simulink model "bici_v2"  (R2013a)
settings: Solver=ode3  SolverMode=SingleTasking  StartTime=0.0  StopTime=10.0  RelTol=1e-3
PreLoadFcn:
  | waijung.modelPreload; % Required for working with Waijung Blockset. Do not remove.
undefined symbols (not defined in the file or in its folder): HSEOSC, Link, LQFP176, ST, STM32F417IG
libraries: simulink x6, stm32f4_tim_lib x6, stm32f4_io_lib x2, stm32f4_adc_lib x1, stm32f4_device_config_lib x1
(part 1 of 2)
CloseFcn:
  | waijung.modelClose; % Required for working with Waijung Blockset. Do not remove.
settings Model: Creator=Juan Esteban  LastModifiedBy=Juan Esteban
settings OptimizationCC: OptimizeModelRefInitCode=on  LifeSpan=1
settings HardwareCC: ProdEndianess=LittleEndian  ProdHWDeviceType=ARM Compatible->Cortex - M4  TargetEndianess=LittleEndian  TargetHWDeviceType=ARM Compatible->Cortex - M4
settings RTWCC: SystemTargetFile=stm32f4.tlc  GenerateMakefile=off  TemplateMakefile=ert_default_tmf  Description=STM32F4 Target  ProcessScript=stm32f4_make_rtw_hook
settings CodeAppCC: IgnoreCustomStorageClasses=off
settings STFCustomTargetCC: ModelReferenceCompliant=off  CombineOutputUpdateFcns=on  ERTCustomFileBanners=on  SupportNonInlinedSFcns=off  MATLABClassNameForMDSCustomization=Simulink.SoftwareTarget.ERTCustomization  SystemTargetFile=stm32f4.tlc
settings ERTTargetCC: GenerateSampleERTMain=off  ModelReferenceCompliant=off  ParMdlRefBuildCompliant=off  CompOptLevelCompliant=off  ConcurrentExecutionCompliant=off  ERTFirstTimeCompliant=off  SupportContinuousTime=on  ModelStepFunctionPrototypeControlCompliant=off  CPPClassGenCompliant=off  ERTSrcFileBannerTemplate=stm32f4_code_template.cgt  ERTHdrFileBannerTemplate=stm32f4_code_template.cgt  ERTDataSrcFileTemplate=stm32f4_code_template.cgt  ERTDataHdrFileTemplate=stm32f4_code_template.cgt  ERTCustomFileTemplate=stm32f4_file_process.tlc

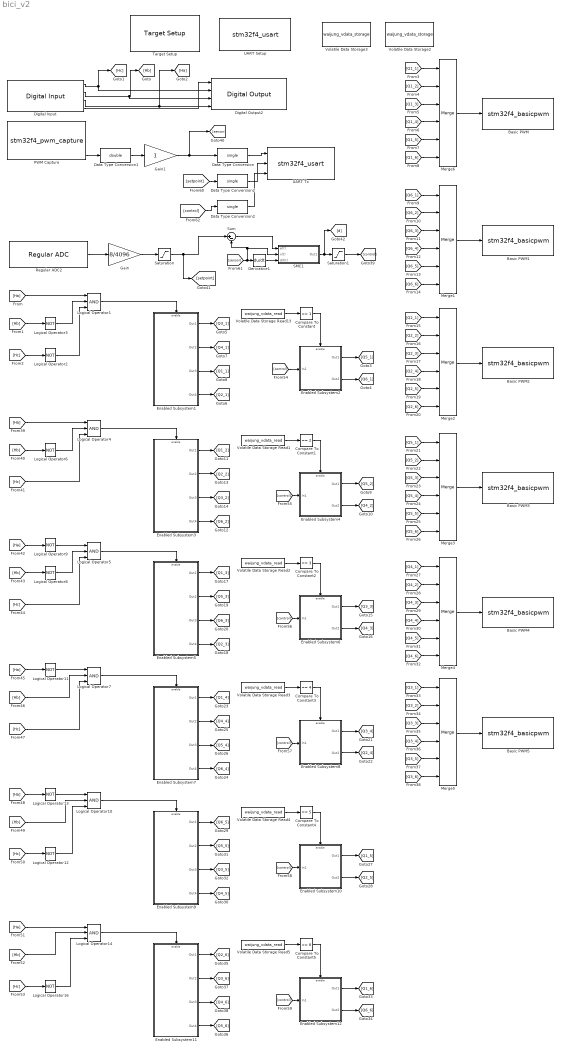
== system bici_v2 ==
  Basic PWM : S-Function  FunctionName=stm32f4_basicpwm  Parameters=timer,pwmperiod,ch1pin,ch2pin,ch3pin,ch4pin,sampletime,sampletimestr,blockid,apb,portstr,pinstr,pinmat,timarr,timprescale,chmat,polaritystr  EnableBusSupport=off  mask(stm32f4_basicpwm){timer=3, pwmperiod=2e-4, polarity=Active High, polaritystr=TIM_OCPolarity_High, ch1pin=A6, ch2pin=Not available - Do not use, ch3pin=Not available - Do not use, ch4pin=Not available - Do not use, sampletime=0.01, sampletimestr=0.01, blockid=BasicPWM, portpinstr=A6,,,, enablecustomportlabel=off, cinputportlabel=In1, In2, In3, In4, coutputportlabel=0, apb=1, portstr=["A"], pinstr=["GPIO_Pin_6"], pinmat=[1 6], timarr=16799, timprescale=0, chmat=[1]}
      mask prompts: pwmperiod "PWM Period (seconds)"; ch1pin "Channel 1"; ch2pin "Channel 2"; ch3pin "Channel 3"; ch4pin "Channel 4"; sampletime "Sample time (sec)"; sampletimestr "Compiled sample time (sec) in string"; portpinstr "Port pin string"; enablecustomportlabel "Enable custom port labels"; cinputportlabel "Custom input port labels (Ex. In1, In2, In3)"; coutputportlabel "Custom output port labels (Ex. Out1, Out2, Out3)"; portstr "Port string"; pinstr "Pin string"; pinmat "Pin matrix"; timarr "Timer ARR"; timprescale "Timer PRESCALE"; chmat "Channel order"
      mask help:
      | This block implements basic Edge-aligned Pulse Width Modulation (PWM) generation.
      | All timers are 16-bit. The PWM period is fixed (per timer).
      mask init:
      | stm32f4_basicpwm_callback('init');
      mask Help: web(fullfile(waijungdocroot,'stm32f4_basicpwm.htm'),'-browser')
      mask TypeOptions timer: 1 | 2 | 3 | 4 | 5 | 8 | 9 | 10 | 11 | 12 | 13 | 14
      mask Callback timer: stm32f4_basicpwm_callback('timer');
      mask Callback pwmperiod: stm32f4_basicpwm_callback('pwmperiod');
      mask TypeOptions polarity: Active High | Active Low
      mask Callback polarity: stm32f4_basicpwm_callback('polarity');
      mask TypeOptions ch1pin: Not available - Do not use | A6 | B4 | C6
      mask Callback ch1pin: stm32f4_basicpwm_callback('ch1pin');
      mask TypeOptions ch2pin: Not available - Do not use | A7 | B5 | C7
      mask Callback ch2pin: stm32f4_basicpwm_callback('ch2pin');
      mask TypeOptions ch3pin: Not available - Do not use | B0 | C8
      mask Callback ch3pin: stm32f4_basicpwm_callback('ch3pin');
      mask TypeOptions ch4pin: Not available - Do not use | B1 | C9
      mask Callback ch4pin: stm32f4_basicpwm_callback('ch4pin');
      mask Callback sampletime: stm32f4_basicpwm_callback('sampletime');
      mask Callback sampletimestr: stm32f4_basicpwm_callback('sampletimestr');
      mask Callback blockid: stm32f4_basicpwm_callback('blockid');
      mask Callback enablecustomportlabel: stm32f4_basicpwm_callback('enablecustomportlabel');
      mask Display: text(0.95, 0.5, 'Timer: 3\nPolarity: Active High\nPeriod (sec) 2e-4\nTs (sec): 0.01','ver','middle','hor','right');port_label('input', 1,'CH1 (A6)')
  Basic PWM1 : S-Function  FunctionName=stm32f4_basicpwm  Parameters=timer,pwmperiod,ch1pin,ch2pin,ch3pin,ch4pin,sampletime,sampletimestr,blockid,apb,portstr,pinstr,pinmat,timarr,timprescale,chmat,polaritystr  EnableBusSupport=off  mask(stm32f4_basicpwm){timer=4, pwmperiod=2e-4, polarity=Active High, polaritystr=TIM_OCPolarity_High, ch1pin=B6, ch2pin=Not available - Do not use, ch3pin=Not available - Do not use, ch4pin=Not available - Do not use, sampletime=0.01, sampletimestr=0.01, blockid=BasicPWM1, portpinstr=B6,,,, enablecustomportlabel=off, cinputportlabel=In1, In2, In3, In4, coutputportlabel=0, apb=1, portstr=["B"], pinstr=["GPIO_Pin_6"], pinmat=[1 6], timarr=16799, timprescale=0, chmat=[1]}
      mask prompts: pwmperiod "PWM Period (seconds)"; ch1pin "Channel 1"; ch2pin "Channel 2"; ch3pin "Channel 3"; ch4pin "Channel 4"; sampletime "Sample time (sec)"; sampletimestr "Compiled sample time (sec) in string"; portpinstr "Port pin string"; enablecustomportlabel "Enable custom port labels"; cinputportlabel "Custom input port labels (Ex. In1, In2, In3)"; coutputportlabel "Custom output port labels (Ex. Out1, Out2, Out3)"; portstr "Port string"; pinstr "Pin string"; pinmat "Pin matrix"; timarr "Timer ARR"; timprescale "Timer PRESCALE"; chmat "Channel order"
      mask help:
      | This block implements basic Edge-aligned Pulse Width Modulation (PWM) generation.
      | All timers are 16-bit. The PWM period is fixed (per timer).
      mask init:
      | stm32f4_basicpwm_callback('init');
      mask Help: web(fullfile(waijungdocroot,'stm32f4_basicpwm.htm'),'-browser')
      mask TypeOptions timer: 1 | 2 | 3 | 4 | 5 | 8 | 9 | 10 | 11 | 12 | 13 | 14
      mask Callback timer: stm32f4_basicpwm_callback('timer');
      mask Callback pwmperiod: stm32f4_basicpwm_callback('pwmperiod');
      mask TypeOptions polarity: Active High | Active Low
      mask Callback polarity: stm32f4_basicpwm_callback('polarity');
      mask TypeOptions ch1pin: Not available - Do not use | B6 | D12
      mask Callback ch1pin: stm32f4_basicpwm_callback('ch1pin');
      mask TypeOptions ch2pin: Not available - Do not use | B7 | D13
      mask Callback ch2pin: stm32f4_basicpwm_callback('ch2pin');
      mask TypeOptions ch3pin: Not available - Do not use | B8 | D14
      mask Callback ch3pin: stm32f4_basicpwm_callback('ch3pin');
      mask TypeOptions ch4pin: Not available - Do not use | B9 | D15
      mask Callback ch4pin: stm32f4_basicpwm_callback('ch4pin');
      mask Callback sampletime: stm32f4_basicpwm_callback('sampletime');
      mask Callback sampletimestr: stm32f4_basicpwm_callback('sampletimestr');
      mask Callback blockid: stm32f4_basicpwm_callback('blockid');
      mask Callback enablecustomportlabel: stm32f4_basicpwm_callback('enablecustomportlabel');
      mask Display: text(0.95, 0.5, 'Timer: 4\nPolarity: Active High\nPeriod (sec) 2e-4\nTs (sec): 0.01','ver','middle','hor','right');port_label('input', 1,'CH1 (B6)')
  Basic PWM2 : S-Function  FunctionName=stm32f4_basicpwm  Parameters=timer,pwmperiod,ch1pin,ch2pin,ch3pin,ch4pin,sampletime,sampletimestr,blockid,apb,portstr,pinstr,pinmat,timarr,timprescale,chmat,polaritystr  EnableBusSupport=off  mask(stm32f4_basicpwm){timer=1, pwmperiod=2e-4, polarity=Active High, polaritystr=TIM_OCPolarity_High, ch1pin=A8, ch2pin=Not available - Do not use, ch3pin=Not available - Do not use, ch4pin=Not available - Do not use, sampletime=0.01, sampletimestr=0.01, blockid=BasicPWM2, portpinstr=A8,,,, enablecustomportlabel=off, cinputportlabel=In1, In2, In3, In4, coutputportlabel=0, apb=2, portstr=["A"], pinstr=["GPIO_Pin_8"], pinmat=[1 8], timarr=33599, timprescale=0, chmat=[1]}
      mask prompts: pwmperiod "PWM Period (seconds)"; ch1pin "Channel 1"; ch2pin "Channel 2"; ch3pin "Channel 3"; ch4pin "Channel 4"; sampletime "Sample time (sec)"; sampletimestr "Compiled sample time (sec) in string"; portpinstr "Port pin string"; enablecustomportlabel "Enable custom port labels"; cinputportlabel "Custom input port labels (Ex. In1, In2, In3)"; coutputportlabel "Custom output port labels (Ex. Out1, Out2, Out3)"; portstr "Port string"; pinstr "Pin string"; pinmat "Pin matrix"; timarr "Timer ARR"; timprescale "Timer PRESCALE"; chmat "Channel order"
      mask help:
      | This block implements basic Edge-aligned Pulse Width Modulation (PWM) generation.
      | All timers are 16-bit. The PWM period is fixed (per timer).
      mask init:
      | stm32f4_basicpwm_callback('init');
      mask Help: web(fullfile(waijungdocroot,'stm32f4_basicpwm.htm'),'-browser')
      mask TypeOptions timer: 1 | 2 | 3 | 4 | 5 | 8 | 9 | 10 | 11 | 12 | 13 | 14
      mask Callback timer: stm32f4_basicpwm_callback('timer');
      mask Callback pwmperiod: stm32f4_basicpwm_callback('pwmperiod');
      mask TypeOptions polarity: Active High | Active Low
      mask Callback polarity: stm32f4_basicpwm_callback('polarity');
      mask TypeOptions ch1pin: Not available - Do not use | A8 | E9
      mask Callback ch1pin: stm32f4_basicpwm_callback('ch1pin');
      mask TypeOptions ch2pin: Not available - Do not use | A9 | E11
      mask Callback ch2pin: stm32f4_basicpwm_callback('ch2pin');
      mask TypeOptions ch3pin: Not available - Do not use | A10 | E13
      mask Callback ch3pin: stm32f4_basicpwm_callback('ch3pin');
      mask TypeOptions ch4pin: Not available - Do not use | A11 | E14
      mask Callback ch4pin: stm32f4_basicpwm_callback('ch4pin');
      mask Callback sampletime: stm32f4_basicpwm_callback('sampletime');
      mask Callback sampletimestr: stm32f4_basicpwm_callback('sampletimestr');
      mask Callback blockid: stm32f4_basicpwm_callback('blockid');
      mask Callback enablecustomportlabel: stm32f4_basicpwm_callback('enablecustomportlabel');
      mask Display: text(0.95, 0.5, 'Timer: 1\nPolarity: Active High\nPeriod (sec) 2e-4\nTs (sec): 0.01','ver','middle','hor','right');port_label('input', 1,'CH1 (A8)')
  Basic PWM3 : S-Function  FunctionName=stm32f4_basicpwm  Parameters=timer,pwmperiod,ch1pin,ch2pin,ch3pin,ch4pin,sampletime,sampletimestr,blockid,apb,portstr,pinstr,pinmat,timarr,timprescale,chmat,polaritystr  EnableBusSupport=off  mask(stm32f4_basicpwm){timer=2, pwmperiod=2e-4, polarity=Active High, polaritystr=TIM_OCPolarity_High, ch1pin=A0, ch2pin=Not available - Do not use, ch3pin=Not available - Do not use, ch4pin=Not available - Do not use, sampletime=0.01, sampletimestr=0.01, blockid=BasicPWM3, portpinstr=A0,,,, enablecustomportlabel=off, cinputportlabel=In1, In2, In3, In4, coutputportlabel=0, apb=1, portstr=["A"], pinstr=["GPIO_Pin_0"], pinmat=[1 0], timarr=16799, timprescale=0, chmat=[1]}
      mask prompts: pwmperiod "PWM Period (seconds)"; ch1pin "Channel 1"; ch2pin "Channel 2"; ch3pin "Channel 3"; ch4pin "Channel 4"; sampletime "Sample time (sec)"; sampletimestr "Compiled sample time (sec) in string"; portpinstr "Port pin string"; enablecustomportlabel "Enable custom port labels"; cinputportlabel "Custom input port labels (Ex. In1, In2, In3)"; coutputportlabel "Custom output port labels (Ex. Out1, Out2, Out3)"; portstr "Port string"; pinstr "Pin string"; pinmat "Pin matrix"; timarr "Timer ARR"; timprescale "Timer PRESCALE"; chmat "Channel order"
      mask help:
      | This block implements basic Edge-aligned Pulse Width Modulation (PWM) generation.
      | All timers are 16-bit. The PWM period is fixed (per timer).
      mask init:
      | stm32f4_basicpwm_callback('init');
      mask Help: web(fullfile(waijungdocroot,'stm32f4_basicpwm.htm'),'-browser')
      mask TypeOptions timer: 1 | 2 | 3 | 4 | 5 | 8 | 9 | 10 | 11 | 12 | 13 | 14
      mask Callback timer: stm32f4_basicpwm_callback('timer');
      mask Callback pwmperiod: stm32f4_basicpwm_callback('pwmperiod');
      mask TypeOptions polarity: Active High | Active Low
      mask Callback polarity: stm32f4_basicpwm_callback('polarity');
      mask TypeOptions ch1pin: Not available - Do not use | A0 | A5 | A15
      mask Callback ch1pin: stm32f4_basicpwm_callback('ch1pin');
      mask TypeOptions ch2pin: Not available - Do not use | A1 | B3
      mask Callback ch2pin: stm32f4_basicpwm_callback('ch2pin');
      mask TypeOptions ch3pin: Not available - Do not use | A2 | B10
      mask Callback ch3pin: stm32f4_basicpwm_callback('ch3pin');
      mask TypeOptions ch4pin: Not available - Do not use | A3 | B11
      mask Callback ch4pin: stm32f4_basicpwm_callback('ch4pin');
      mask Callback sampletime: stm32f4_basicpwm_callback('sampletime');
      mask Callback sampletimestr: stm32f4_basicpwm_callback('sampletimestr');
      mask Callback blockid: stm32f4_basicpwm_callback('blockid');
      mask Callback enablecustomportlabel: stm32f4_basicpwm_callback('enablecustomportlabel');
      mask Display: text(0.95, 0.5, 'Timer: 2\nPolarity: Active High\nPeriod (sec) 2e-4\nTs (sec): 0.01','ver','middle','hor','right');port_label('input', 1,'CH1 (A0)')
  Basic PWM4 : S-Function  FunctionName=stm32f4_basicpwm  Parameters=timer,pwmperiod,ch1pin,ch2pin,ch3pin,ch4pin,sampletime,sampletimestr,blockid,apb,portstr,pinstr,pinmat,timarr,timprescale,chmat,polaritystr  EnableBusSupport=off  mask(stm32f4_basicpwm){timer=5, pwmperiod=2e-4, polarity=Active High, polaritystr=TIM_OCPolarity_High, ch1pin=Not available - Do not use, ch2pin=A1, ch3pin=Not available - Do not use, ch4pin=Not available - Do not use, sampletime=0.01, sampletimestr=0.01, blockid=BasicPWM4, portpinstr=,A1,,, enablecustomportlabel=off, cinputportlabel=In1, In2, In3, In4, coutputportlabel=0, apb=1, portstr=["A"], pinstr=["GPIO_Pin_1"], pinmat=[1 1], timarr=16799, timprescale=0, chmat=[2]}
      mask prompts: pwmperiod "PWM Period (seconds)"; ch1pin "Channel 1"; ch2pin "Channel 2"; ch3pin "Channel 3"; ch4pin "Channel 4"; sampletime "Sample time (sec)"; sampletimestr "Compiled sample time (sec) in string"; portpinstr "Port pin string"; enablecustomportlabel "Enable custom port labels"; cinputportlabel "Custom input port labels (Ex. In1, In2, In3)"; coutputportlabel "Custom output port labels (Ex. Out1, Out2, Out3)"; portstr "Port string"; pinstr "Pin string"; pinmat "Pin matrix"; timarr "Timer ARR"; timprescale "Timer PRESCALE"; chmat "Channel order"
      mask help:
      | This block implements basic Edge-aligned Pulse Width Modulation (PWM) generation.
      | All timers are 16-bit. The PWM period is fixed (per timer).
      mask init:
      | stm32f4_basicpwm_callback('init');
      mask Help: web(fullfile(waijungdocroot,'stm32f4_basicpwm.htm'),'-browser')
      mask TypeOptions timer: 1 | 2 | 3 | 4 | 5 | 8 | 9 | 10 | 11 | 12 | 13 | 14
      mask Callback timer: stm32f4_basicpwm_callback('timer');
      mask Callback pwmperiod: stm32f4_basicpwm_callback('pwmperiod');
      mask TypeOptions polarity: Active High | Active Low
      mask Callback polarity: stm32f4_basicpwm_callback('polarity');
      mask TypeOptions ch1pin: Not available - Do not use | A0 | H10
      mask Callback ch1pin: stm32f4_basicpwm_callback('ch1pin');
      mask TypeOptions ch2pin: Not available - Do not use | A1 | H11
      mask Callback ch2pin: stm32f4_basicpwm_callback('ch2pin');
      mask TypeOptions ch3pin: Not available - Do not use | A2 | H12
      mask Callback ch3pin: stm32f4_basicpwm_callback('ch3pin');
      mask TypeOptions ch4pin: Not available - Do not use | A3 | I0
      mask Callback ch4pin: stm32f4_basicpwm_callback('ch4pin');
      mask Callback sampletime: stm32f4_basicpwm_callback('sampletime');
      mask Callback sampletimestr: stm32f4_basicpwm_callback('sampletimestr');
      mask Callback blockid: stm32f4_basicpwm_callback('blockid');
      mask Callback enablecustomportlabel: stm32f4_basicpwm_callback('enablecustomportlabel');
      mask Display: text(0.95, 0.5, 'Timer: 5\nPolarity: Active High\nPeriod (sec) 2e-4\nTs (sec): 0.01','ver','middle','hor','right');port_label('input', 1,'CH2 (A1)')
  Basic PWM5 : S-Function  FunctionName=stm32f4_basicpwm  Parameters=timer,pwmperiod,ch1pin,ch2pin,ch3pin,ch4pin,sampletime,sampletimestr,blockid,apb,portstr,pinstr,pinmat,timarr,timprescale,chmat,polaritystr  EnableBusSupport=off  mask(stm32f4_basicpwm){timer=9, pwmperiod=2e-4, polarity=Active High, polaritystr=TIM_OCPolarity_High, ch1pin=A2, ch2pin=Not available - Do not use, ch3pin=Not available - Do not use, ch4pin=Not available - Do not use, sampletime=0.01, sampletimestr=0.01, blockid=BasicPWM5, portpinstr=A2,,,, enablecustomportlabel=off, cinputportlabel=In1, In2, In3, In4, coutputportlabel=0, apb=2, portstr=["A"], pinstr=["GPIO_Pin_2"], pinmat=[1 2], timarr=33599, timprescale=0, chmat=[1]}
      mask prompts: pwmperiod "PWM Period (seconds)"; ch1pin "Channel 1"; ch2pin "Channel 2"; ch3pin "Channel 3"; ch4pin "Channel 4"; sampletime "Sample time (sec)"; sampletimestr "Compiled sample time (sec) in string"; portpinstr "Port pin string"; enablecustomportlabel "Enable custom port labels"; cinputportlabel "Custom input port labels (Ex. In1, In2, In3)"; coutputportlabel "Custom output port labels (Ex. Out1, Out2, Out3)"; portstr "Port string"; pinstr "Pin string"; pinmat "Pin matrix"; timarr "Timer ARR"; timprescale "Timer PRESCALE"; chmat "Channel order"
      mask help:
      | This block implements basic Edge-aligned Pulse Width Modulation (PWM) generation.
      | All timers are 16-bit. The PWM period is fixed (per timer).
      mask init:
      | stm32f4_basicpwm_callback('init');
      mask Help: web(fullfile(waijungdocroot,'stm32f4_basicpwm.htm'),'-browser')
      mask TypeOptions timer: 1 | 2 | 3 | 4 | 5 | 8 | 9 | 10 | 11 | 12 | 13 | 14
      mask Callback timer: stm32f4_basicpwm_callback('timer');
      mask Callback pwmperiod: stm32f4_basicpwm_callback('pwmperiod');
      mask TypeOptions polarity: Active High | Active Low
      mask Callback polarity: stm32f4_basicpwm_callback('polarity');
      mask TypeOptions ch1pin: Not available - Do not use | A2 | E5
      mask Callback ch1pin: stm32f4_basicpwm_callback('ch1pin');
      mask TypeOptions ch2pin: Not available - Do not use | A3 | E6
      mask Callback ch2pin: stm32f4_basicpwm_callback('ch2pin');
      mask TypeOptions ch3pin: Not available - Do not use
      mask Callback ch3pin: stm32f4_basicpwm_callback('ch3pin');
      mask TypeOptions ch4pin: Not available - Do not use
      mask Callback ch4pin: stm32f4_basicpwm_callback('ch4pin');
      mask Callback sampletime: stm32f4_basicpwm_callback('sampletime');
      mask Callback sampletimestr: stm32f4_basicpwm_callback('sampletimestr');
      mask Callback blockid: stm32f4_basicpwm_callback('blockid');
      mask Callback enablecustomportlabel: stm32f4_basicpwm_callback('enablecustomportlabel');
      mask Display: text(0.95, 0.5, 'Timer: 9\nPolarity: Active High\nPeriod (sec) 2e-4\nTs (sec): 0.01','ver','middle','hor','right');port_label('input', 1,'CH1 (A2)')
  Compare To Constant : simulink/Logic and Bit Operations/Compare To Constant  relop===  const=1  OutDataTypeStr=boolean
  Compare To Constant1 : simulink/Logic and Bit Operations/Compare To Constant  relop===  const=2  OutDataTypeStr=boolean
  Compare To Constant2 : simulink/Logic and Bit Operations/Compare To Constant  relop===  const=3  OutDataTypeStr=boolean
  Compare To Constant3 : simulink/Logic and Bit Operations/Compare To Constant  relop===  const=4  OutDataTypeStr=boolean
  Compare To Constant4 : simulink/Logic and Bit Operations/Compare To Constant  relop===  const=5  OutDataTypeStr=boolean
  Compare To Constant5 : simulink/Logic and Bit Operations/Compare To Constant  relop===  const=6  OutDataTypeStr=boolean
  Data Type Conversion : DataTypeConversion  OutDataTypeStr=single
  Data Type Conversion1 : DataTypeConversion  OutDataTypeStr=double
  Data Type Conversion2 : DataTypeConversion  OutDataTypeStr=single
  "Data Type Conversion2 " : DataTypeConversion  OutDataTypeStr=single
  Derivative1 : Derivative  CoefficientInTFapproximation=0
  Digital Input : stm32f4_io_lib/Digital Input  port=D  speed=100  porttype=Pull Up  porttypestr=UP  use_pin0=on  use_pin1=on  use_pin2=on  use_pin3=on  use_pin4=off  use_pin5=off  use_pin6=off  use_pin7=off  use_pin8=off  use_pin9=off  use_pin10=off  use_pin11=off  use_pin12=off  use_pin13=off  use_pin14=off  use_pin15=off  pinstr=GPIO_Pin_0 | GPIO_Pin_1 | GPIO_Pin_2 | GPIO_Pin_3  usedpinarray="[1  1  1  1  0  0  0  0  0  0  0  0  0  0  0  0]"  bitbandingstr=|  sampletime=-1  sampletimestr=0.01  blockid=DigitalInput  enablecustomportlabel=off  glabalinit=off  cinputportlabel=In1, In2  coutputportlabel=Out1, Out2
      | #define DigitalInput_D0 Peripheral_BB(GPIOD->IDR, 0)  /* Output pin */
      | #define DigitalInput_D1 Peripheral_BB(GPIOD->IDR, 1)  /* Output pin */
      | #define DigitalInput_D2 Peripheral_BB(GPIOD->IDR, 2)  /* Output pin */
      | #define DigitalInput_D3 Peripheral_BB(GPIOD->IDR, 3)  /* Output pin */
  Digital Output2 : stm32f4_io_lib/Digital Output  use_bitband=on  port=D  speed=100  porttype=Push Pull  porttypestr=PP  use_pin0=off  use_pin1=off  use_pin2=off  use_pin3=off  use_pin4=off  use_pin5=off  use_pin6=off  use_pin7=off  use_pin8=off  use_pin9=off  use_pin10=off  use_pin11=off  use_pin12=on  use_pin13=on  use_pin14=on  use_pin15=on  pinstr=GPIO_Pin_12 | GPIO_Pin_13 | GPIO_Pin_14 | GPIO_Pin_15  usedpinarray="[0  0  0  0  0  0  0  0  0  0  0  0  1  1  1  1]"  bitbandingstr=|  sampletime=-1  sampletimestr=0.01  blockid=DigitalOutput2  enablecustomportlabel=off  globalinit=off  cinputportlabel=In1, In2  coutputportlabel=0
      | #define DigitalOutput2_D12 Peripheral_BB(GPIOD->ODR, 12)  /* Output pin */
      | #define DigitalOutput2_D13 Peripheral_BB(GPIOD->ODR, 13)  /* Output pin */
      | #define DigitalOutput2_D14 Peripheral_BB(GPIOD->ODR, 14)  /* Output pin */
      | #define DigitalOutput2_D15 Peripheral_BB(GPIOD->ODR, 15)  /* Output pin */
  Enabled Subsystem1 : Subsystem  TreatAsAtomicUnit=on
  Enabled Subsystem10 : Subsystem  TreatAsAtomicUnit=on
  Enabled Subsystem11 : Subsystem  TreatAsAtomicUnit=on
  Enabled Subsystem12 : Subsystem  TreatAsAtomicUnit=on
  Enabled Subsystem2 : Subsystem  TreatAsAtomicUnit=on
  Enabled Subsystem3 : Subsystem  TreatAsAtomicUnit=on
  Enabled Subsystem4 : Subsystem  TreatAsAtomicUnit=on
  Enabled Subsystem5 : Subsystem  TreatAsAtomicUnit=on
  Enabled Subsystem6 : Subsystem  TreatAsAtomicUnit=on
  Enabled Subsystem7 : Subsystem  TreatAsAtomicUnit=on
  Enabled Subsystem8 : Subsystem  TreatAsAtomicUnit=on
  Enabled Subsystem9 : Subsystem  TreatAsAtomicUnit=on
  Gain : Gain  Gain=8/4096
  Gain1 : Gain
  Logical Operator{1,4..5,7,10,14} (6 alike) : Logic  Inputs=3  AllPortsSameDT=off  OutDataTypeStr=boolean
  Logical Operator{2..3,6,8..9,11..13,16} (9 alike) : Logic  Operator=NOT  Inputs=3  AllPortsSameDT=off  OutDataTypeStr=boolean
  Merge{1..6} (6 alike) : Merge  Inputs=6
  PWM Capture : S-Function  FunctionName=stm32f4_pwm_capture  Parameters=conf,inputporttype,inputportwidth,outputporttype,outputportwidth,optionstring,sampletime,blockid  EnableBusSupport=off  mask(stm32f4_pwm_capture){conf=Capture, timer=8, lasttimer=8, pin=C7, pintype=Pull Up, edge=Rising, datatype=single, portpinstr=0, sampletime=inf, blockid=PWMCapture, inputporttype=[], inputportwidth=[], inputportlabel={}, outputporttype=[3 1 1 1], outputportwidth=[], outputportlabel={'READY','+Width (sec)','+Duty (%)','Frequency (Hz)'}, compat=0, optionstring=["8","2","C","7","2","16","Rising","UP","float"]}
      mask prompts: conf "Configuration"; lasttimer "Last Timer"; pin "Capture Pin"; pintype "Capture Pin Type (Pull-Up/Pull-Down)"; edge "Capture Edge"; datatype "Output data type"; portpinstr "Port Pin String"; sampletime "Sample time (sec)"; blockid "Block ID"; inputporttype "Input Port Type"; inputportwidth "Input Port Width"; inputportlabel "Input Port Label"; outputporttype "Output Port Type"; outputportwidth "Output Port Width"; outputportlabel "Output port label"; compat "Compatibility (Reserved for future use)"; optionstring "String(s) to be passed to TLC"
      mask help:
      | Capture Edge:
      |  Rising - PWM period start from rising edge of pulse N to rising edge of pulse N+1
      |  Falling - PWM period start from falling edge of pulse N to falling edge of pulse N+1
      | Capture data type:
      |  Capture data type, selectable to double or single.
      |
      | Output:
      |  READY - indicate the status of capture, a non-zero value indicate data is ready.
      |  +Width - positive pulse width, in unit of second.
      |  +Duty - positive duty cycle, 0 to 100%
      |  Frequency - signal frequency in unit of Hz
      |
      | Note: caprure period should not longer than 1 second (Maximum limit is 3 seconds)
      mask init:
      | stm32f4_pwm_capture_callback('init');
      mask Help: web(fullfile(waijungdocroot,'stm32f4_pwm_capture.htm'), '-browser')
      mask TypeOptions conf: Capture
      mask Callback conf: stm32f4_pwm_capture_callback('conf');
      mask TypeOptions timer: 1 | 2 | 3 | 4 | 5 | 8
      mask Callback timer: stm32f4_pwm_capture_callback('timer');
      mask TypeOptions pin: Not used | C6 | I5 | C7 | I6 | C8 | I7 | C9 | I2
      mask TypeOptions pintype: None | Pull Up | Pull Down
      mask TypeOptions edge: Rising | Falling
      mask TypeOptions datatype: double | single
      mask Callback sampletime: stm32f4_pwm_capture_callback('sampletime');
      mask Callback blockid: stm32f4_pwm_capture_callback('blockid');
      mask Display: text(0.05, 0.5, 'Timer: 8 (16 bit)\nInput Pin: C7\nEdge: Rising\nTs (sec): 0.01','ver','middle','hor','left'); port_label('output', 1,'READY'); port_label('output', 2,'+Width (sec)'); port_label('output', 3,'+Duty (%)'); port_label('output', 4,'Frequency (Hz)');
  Regular ADC2 : stm32f4_adc_lib/Regular ADC  adcmodule=1  outputdatatype=Double  prescaler=2  prescalerstr=ADC_Prescaler_Div2  chsamplingtime=Auto  chsamplingtimestr=ADC_SampleTime_480Cycles  read_an0=off  read_an1=off  read_an2=off  read_an3=off  read_an4=off  read_an5=off  read_an6=off  read_an7=off  read_an8=off  read_an9=off  read_an10=on  read_an11=off  read_an12=off  read_an13=off  read_an14=off  read_an15=off  read_an16=off  read_an17=off  read_an18=off  pinstr=GPIO_Pin_10  usedpinarray="[0  0  0  0  0  0  0  0  0  0  1  0  0  0  0  0  0  0  0]"  usedportidarray=[2]  usedpinidarray=[0]  usedpinidcount=1  sampletime=-1  blockid=RegularADC2  enablecustomportlabel=off  cinputportlabel=0  coutputportlabel=Out1, Out2
  SMC1 : Subsystem  TreatAsAtomicUnit=on
  Saturation : Saturate  UpperLimit=8  LowerLimit=0
  Saturation1 : Saturate  UpperLimit=60  LowerLimit=0
  Sum : Sum  Inputs=|+-
  Target Setup : stm32f4_device_config_lib/Target Setup  Priority=100  compiler=GNU ARM  previous_compiler=GNU ARM  mcu=STM32F417IG (LQFP176)  mcustr=STM32F417IG  clockconfig=HSEOSC-8MHz  system_stm32f4xx_c_path=C:\waijung17_03a\targets\stm32f4_target\stm32f4\utils\system_stm32f4xx_default\STM32F40_41xxx\hseosc8mhz  showmemoryconfiguration=off  stacksize=0x2000  heapsize=0x2000  enableautocompiledownload=on  fullchiperase=on  programmerinterface=ST-Link  editctrlstr=on  compilercontrolstr=$(patsubst %, -I%, .) -mcpu=cortex-m4 -mthumb -mthumb-interwork -mfloat-abi=hard -mfpu=fpv4-sp-d16 -ffast-math -Wall -Wextra -Ofast  assemblercontrolstr=$(patsubst %, -I%, .) -mcpu=cortex-m4 -mthumb -mthumb-interwork -mfloat-abi=hard -mfpu=fpv4-sp-d16 -ffast-math -Wall -Wextra -Ofast -Wa,-amhls=$(<:.s=.lst) -D__STACK_SIZE=$(STACK_SIZE) -D__HEAP_SIZE=$(HEAP_SIZE)  linkercontrolstr=-T$(LD_SCRIPT) -g -Wl,-Map=$(MAP),--cref,--no-warn-mismatch -mcpu=cortex-m4 -mthumb -mthumb-interwork -mfloat-abi=hard -mfpu=fpv4-sp-d16 -specs=nosys.specs  runafterdownload=on  execprofile=None  profileruart=3  profilerbaud=500000  profilertxpin=D8  profilerinitstr=0.01,168000000,1680000,500000,0  manualsetsampletime=off  sampletime=0.01  blockid=TargetSetup  systickreloadvalue=1680000  hseval=8000000  lastprofileruart=3  hclk=168000000  flashorigin=0x8000000  flashlength=1024k  ramorigin=0x20000000  ramlength=128k  useextram=off
  UART Setup : S-Function  Priority=1  FunctionName=stm32f4_usart  Parameters=configuration,uartmodule,transfer,baudrate,inputtype,outputtype,confstr,binheaderarray,binterminatorarray,asciiheader,asciiterminator,bindatalength,packetmode,varname,sampletime,sampletimestr,blockid  EnableBusSupport=off  mask(stm32f4_usart){configuration=Setup, uartmodule=3, baudrate=115200, databits=8, parity=No, stopbit=1, remaptxpin=D8, remaprxpin=D9, flowcontrol=None, remapctspin=Not used, remaprtspin=Not used, advanceoptions=off, rxbuffersize=512, txbuffersize=512, transfer=Blocking, packetmode=Ascii, binheader='7E 7E', binterminator='03 03', porttype_double=1, porttype_single=0, porttype_int8=1, porttype_uint8=0, porttype_int16=0, porttype_uint16=0, porttype_int32=0, porttype_uint32=0, asciiformat='%d,%f', rx_asciiterminator=CRLF (0x0D 0x0A - "\r\n"), tx_asciiterminator=CR (0x0D - "\r"), storagename=<empty>, varname=, inputtype=[0], outputtype=[0], binheaderarray=[0], binterminatorarray=[0], bindatalength=0, asciiheader='', asciiterminator=[0], sampletime=-1, sampletimestr=0.01, blockid=UARTSetup, confstr=[ "dummy", "1", "D", "8", "1", "D", "9", "0", "*", "*", "0", "*", "*", "1", "4", "3", "1", "4", "1", "512", "512", "1", "3", "115200", "8", "No", "1", "None", "USART3"], lastmodule=3}
      mask prompts: uartmodule "UART Module"; baudrate "Baud rate (bps)"; databits "Data bits"; stopbit "Stop bit"; remaptxpin "Tx Pin"; remaprxpin "Rx Pin"; flowcontrol "Hardware flow control"; remapctspin "HW Flow control, CTS Pin"; remaprtspin "HW Flow control, RTS Pin"; advanceoptions "Advance options"; rxbuffersize "Rx buffer size (bytes)"; txbuffersize "Tx buffer size (bytes)"; packetmode "Packet mode"; binheader "Binary header (example: '7E 7E')"; binterminator "Binary terminator (example: '03 03')"; porttype_double "Number of data port, type DOUBLE"; porttype_single "Number of data port, type SINGLE"; porttype_int8 "Number of data port, type INT8"; porttype_uint8 "Number of data port, type UINT8"; porttype_int16 "Number of data port, type INT16"; porttype_uint16 "Number of data port, type UINT16"; porttype_int32 "Number of data port, type INT32"; porttype_uint32 "Number of data port, type UINT32"; asciiformat "Ascii format"; rx_asciiterminator "End of packet"; tx_asciiterminator "End of packet"; storagename "Buffer"; varname "Var name"; inputtype "Input data type"; outputtype "Output data type"; binheaderarray "Binary header"; binterminatorarray "Binary terminator"; bindatalength "Binary data length"; asciiheader "Ascii header (printf format)"; asciiterminator "Ascii terminator"; sampletime "Sample time (sec)"; sampletimestr "Compiled sample time (sec) in string"; confstr "Configuration string"; lastmodule "Last module selected"
      mask init:
      | stm32f4_usart_callback('init');
      mask Help: web(fullfile(waijungdocroot,'stm32f4_usart_setup.htm'), '-browser')
      mask TypeOptions configuration: Setup | Tx | Rx
      mask Callback configuration: stm32f4_usart_callback('configuration');
      mask TypeOptions uartmodule: 1 | 2 | 3 | 4 | 5 | 6
      mask Callback uartmodule: stm32f4_usart_callback('uartmodule');
      mask Callback baudrate: stm32f4_usart_callback('baudrate');
      mask TypeOptions databits: 8
      mask TypeOptions parity: No | Odd | Even
      mask TypeOptions stopbit: 0.5 | 1 | 1.5 | 2
      mask TypeOptions remaptxpin: Not used | B10 | C10 | D8
      mask TypeOptions remaprxpin: Not used | B11 | C11 | D9
      mask TypeOptions flowcontrol: None | RTS | CTS | RTS/CTS
      mask Callback flowcontrol: stm32f4_usart_callback('flowcontrol');
      mask TypeOptions remapctspin: Not used | B13 | D11
      mask TypeOptions remaprtspin: Not used | B14 | D12
      mask Callback advanceoptions: stm32f4_usart_callback('advanceoptions');
      mask TypeOptions rxbuffersize: 16 | 32 | 64 | 128 | 256 | 512 | 1024 | 2048
      mask TypeOptions txbuffersize: 16 | 32 | 64 | 128 | 256 | 512 | 1024 | 2048
      mask TypeOptions transfer: Blocking | Non-Blocking
      mask Callback transfer: stm32f4_usart_callback('transfer');
      mask TypeOptions packetmode: Ascii | Binary | String Buffer
      mask Callback packetmode: stm32f4_usart_callback('packetmode');
      mask Callback binheader: stm32f4_usart_callback('binheader');
      mask Callback binterminator: stm32f4_usart_callback('binterminator');
      mask Callback porttype_double: stm32f4_usart_callback('porttype');
      mask Callback porttype_single: stm32f4_usart_callback('porttype');
      mask Callback porttype_int8: stm32f4_usart_callback('porttype');
      mask Callback porttype_uint8: stm32f4_usart_callback('porttype');
      mask Callback porttype_int16: stm32f4_usart_callback('porttype');
      mask Callback porttype_uint16: stm32f4_usart_callback('porttype');
      mask Callback porttype_int32: stm32f4_usart_callback('porttype');
      mask Callback porttype_uint32: stm32f4_usart_callback('porttype');
      mask Callback asciiformat: stm32f4_usart_callback('asciiformat');
      mask TypeOptions rx_asciiterminator: CR (0x0D - "\r") | LF (0x0A - "\n") | CRLF (0x0D 0x0A - "\r\n")
      mask Callback rx_asciiterminator: stm32f4_usart_callback('rx_asciiterminator');
      mask TypeOptions tx_asciiterminator: CR (0x0D - "\r") | LF (0x0A - "\n") | CRLF (0x0D 0x0A - "\r\n") | None
      mask Callback tx_asciiterminator: stm32f4_usart_callback('tx_asciiterminator');
      mask TypeOptions storagename: <empty>
      mask Callback storagename: stm32f4_usart_callback('storagename');
      mask Callback varname: stm32f4_usart_callback('varname');
      mask Callback sampletime: stm32f4_usart_callback('sampletime');
      mask Callback sampletimestr: stm32f4_usart_callback('sampletimestr');
      mask Callback blockid: stm32f4_usart_callback('blockid');
      mask Display: text(0.5, 0.5, 'Module: USART3_Setup\nBaud (Bps): 115200\nDMA Buffer: 512/512\nTx/Rx Pin: D8/D9','ver','middle','hor','center');
  UART Tx : S-Function  Priority=1  FunctionName=stm32f4_usart  Parameters=configuration,uartmodule,transfer,baudrate,inputtype,outputtype,confstr,binheaderarray,binterminatorarray,asciiheader,asciiterminator,bindatalength,packetmode,varname,sampletime,sampletimestr,blockid  EnableBusSupport=off  mask(stm32f4_usart){configuration=Tx, uartmodule=3, baudrate=115200, databits=8, parity=No, stopbit=1, remaptxpin=Not used, remaprxpin=Not used, flowcontrol=None, remapctspin=Not used, remaprtspin=Not used, advanceoptions=off, rxbuffersize=512, txbuffersize=512, transfer=Blocking, packetmode=Ascii, binheader='7E 7E', binterminator='03 03', porttype_double=1, porttype_single=0, porttype_int8=1, porttype_uint8=0, porttype_int16=0, porttype_uint16=0, porttype_int32=0, porttype_uint32=0, asciiformat='%f,%f,%f', rx_asciiterminator=CRLF (0x0D 0x0A - "\r\n"), tx_asciiterminator=CR (0x0D - "\r"), storagename=<empty>, varname=, inputtype=[3  1 1 1], outputtype=[0], binheaderarray=[0], binterminatorarray=[0], bindatalength=0, asciiheader='%f,%f,%f\r', asciiterminator=[1 13], sampletime=-1, sampletimestr=0, blockid=UARTTx, confstr=[ "dummy", "0", "*", "*", "0", "*", "*", "0", "*", "*", "0", "*", "*", "1", "4", "3", "1", "4", "1", "512", "512", "1", "3", "115200", "8", "No", "1", "None", "USART3"], lastmodule=1}
      mask prompts: uartmodule "UART Module"; baudrate "Baud rate (bps)"; databits "Data bits"; stopbit "Stop bit"; remaptxpin "Tx Pin"; remaprxpin "Rx Pin"; flowcontrol "Hardware flow control"; remapctspin "HW Flow control, CTS Pin"; remaprtspin "HW Flow control, RTS Pin"; advanceoptions "Advance options"; rxbuffersize "Rx buffer size (bytes)"; txbuffersize "Tx buffer size (bytes)"; packetmode "Packet mode"; binheader "Binary header (example: '7E 7E')"; binterminator "Binary terminator (example: '03 03')"; porttype_double "Number of data port, type DOUBLE"; porttype_single "Number of data port, type SINGLE"; porttype_int8 "Number of data port, type INT8"; porttype_uint8 "Number of data port, type UINT8"; porttype_int16 "Number of data port, type INT16"; porttype_uint16 "Number of data port, type UINT16"; porttype_int32 "Number of data port, type INT32"; porttype_uint32 "Number of data port, type UINT32"; asciiformat "Ascii format"; rx_asciiterminator "End of packet"; tx_asciiterminator "End of packet"; storagename "Buffer"; varname "Var name"; inputtype "Input data type"; outputtype "Output data type"; binheaderarray "Binary header"; binterminatorarray "Binary terminator"; bindatalength "Binary data length"; asciiheader "Ascii header (printf format)"; asciiterminator "Ascii terminator"; sampletime "Sample time (sec)"; sampletimestr "Compiled sample time (sec) in string"; confstr "Configuration string"; lastmodule "Last module selected"
      mask help:
      | Data type for Ascii format
      | %u, %i, %d, %o, %x: uint32
      | %e, %g, %f: single
      | %c: int8
      mask init:
      | stm32f4_usart_callback('init');
      mask Help: web(fullfile(waijungdocroot,'stm32f4_usart_tx.htm'), '-browser')
      mask TypeOptions configuration: Setup | Tx | Rx
      mask Callback configuration: stm32f4_usart_callback('configuration');
      mask TypeOptions uartmodule: 1 | 2 | 3 | 4 | 5 | 6
      mask Callback uartmodule: stm32f4_usart_callback('uartmodule');
      mask Callback baudrate: stm32f4_usart_callback('baudrate');
      mask TypeOptions databits: 8
      mask TypeOptions parity: No | Odd | Even
      mask TypeOptions stopbit: 0.5 | 1 | 1.5 | 2
      mask TypeOptions remaptxpin: Not used | A9 | B6
      mask TypeOptions remaprxpin: Not used | A10 | B7
      mask TypeOptions flowcontrol: None | RTS | CTS | RTS/CTS
      mask Callback flowcontrol: stm32f4_usart_callback('flowcontrol');
      mask TypeOptions remapctspin: Not used | A11
      mask TypeOptions remaprtspin: Not used | A12
      mask Callback advanceoptions: stm32f4_usart_callback('advanceoptions');
      mask TypeOptions rxbuffersize: 16 | 32 | 64 | 128 | 256 | 512 | 1024 | 2048
      mask TypeOptions txbuffersize: 16 | 32 | 64 | 128 | 256 | 512 | 1024 | 2048
      mask TypeOptions transfer: Blocking | Non-Blocking
      mask Callback transfer: stm32f4_usart_callback('transfer');
      mask TypeOptions packetmode: Ascii | Binary | Binary Vector | String Buffer | Raw Buffer
      mask Callback packetmode: stm32f4_usart_callback('packetmode');
      mask Callback binheader: stm32f4_usart_callback('binheader');
      mask Callback binterminator: stm32f4_usart_callback('binterminator');
      mask Callback porttype_double: stm32f4_usart_callback('porttype');
      mask Callback porttype_single: stm32f4_usart_callback('porttype');
      mask Callback porttype_int8: stm32f4_usart_callback('porttype');
      mask Callback porttype_uint8: stm32f4_usart_callback('porttype');
      mask Callback porttype_int16: stm32f4_usart_callback('porttype');
      mask Callback porttype_uint16: stm32f4_usart_callback('porttype');
      mask Callback porttype_int32: stm32f4_usart_callback('porttype');
      mask Callback porttype_uint32: stm32f4_usart_callback('porttype');
      mask Callback asciiformat: stm32f4_usart_callback('asciiformat');
      mask TypeOptions rx_asciiterminator: CR (0x0D - "\r") | LF (0x0A - "\n") | CRLF (0x0D 0x0A - "\r\n")
      mask Callback rx_asciiterminator: stm32f4_usart_callback('rx_asciiterminator');
      mask TypeOptions tx_asciiterminator: CR (0x0D - "\r") | LF (0x0A - "\n") | CRLF (0x0D 0x0A - "\r\n") | None
      mask Callback tx_asciiterminator: stm32f4_usart_callback('tx_asciiterminator');
      mask TypeOptions storagename: <empty>
      mask Callback storagename: stm32f4_usart_callback('storagename');
      mask Callback varname: stm32f4_usart_callback('varname');
      mask Callback sampletime: stm32f4_usart_callback('sampletime');
      mask Callback sampletimestr: stm32f4_usart_callback('sampletimestr');
      mask Callback blockid: stm32f4_usart_callback('blockid');
      mask Display: text(0.95, 0.5, 'Module: USART3_Tx\nPacket: Ascii\nTransfer: Blocking\nTs (sec): 0','ver','middle','hor','right'); port_label('input', 1,'single'); port_label('input', 2,'single'); port_label('input', 3,'single');
  Volatile Data Storage Read1 : S-Function  FunctionName=waijung_vdata_read  Parameters=storagename,varname,sampletime,sampletimestr,blockid,storagetype,storagetypestr  EnableBusSupport=off  mask(waijung_vdata_read){storagename=c, varname=VolatileDataStorage3_c, sampletime=-1, sampletimestr=0.01, blockid=VolatileDataStorageRead1, storagetype=double, storagetypestr=double}
      mask prompts: storagename "Storage Name"; varname "Variable name"; sampletime "Sample time (sec)"; sampletimestr "Compiled sample time (sec) in string"; storagetype "Data type"; storagetypestr "Data type string"
      mask help: This block implements read data from a buffer.
      mask init:
      | waijung_vdata_read_callback('init');
      mask Help: web(fullfile(waijungdocroot,'Volatile_Data_Storage_Read.htm'))
      mask TypeOptions storagename: condicion | c
      mask Callback storagename: waijung_vdata_read_callback('storagename');
      mask Callback varname: waijung_vdata_read_callback('varname');
      mask Callback sampletime: waijung_vdata_read_callback('sampletime');
      mask Callback sampletimestr: waijung_vdata_read_callback('sampletimestr');
      mask Callback blockid: waijung_vdata_read_callback('blockid');
      mask Callback storagetype: waijung_vdata_read_callback('storagetype');
      mask Display: text(0.05, 0.5, 'Buffer: c','ver','middle','hor','left');port_label('output',1,'D1(double)')
  Volatile Data Storage Read13 : S-Function  FunctionName=waijung_vdata_read  Parameters=storagename,varname,sampletime,sampletimestr,blockid,storagetype,storagetypestr  EnableBusSupport=off  mask(waijung_vdata_read){storagename=c, varname=VolatileDataStorage3_c, sampletime=-1, sampletimestr=0.01, blockid=VolatileDataStorageRead13, storagetype=double, storagetypestr=double}
      mask prompts: storagename "Storage Name"; varname "Variable name"; sampletime "Sample time (sec)"; sampletimestr "Compiled sample time (sec) in string"; storagetype "Data type"; storagetypestr "Data type string"
      mask help: This block implements read data from a buffer.
      mask init:
      | waijung_vdata_read_callback('init');
      mask Help: web(fullfile(waijungdocroot,'Volatile_Data_Storage_Read.htm'))
      mask TypeOptions storagename: condicion | c
      mask Callback storagename: waijung_vdata_read_callback('storagename');
      mask Callback varname: waijung_vdata_read_callback('varname');
      mask Callback sampletime: waijung_vdata_read_callback('sampletime');
      mask Callback sampletimestr: waijung_vdata_read_callback('sampletimestr');
      mask Callback blockid: waijung_vdata_read_callback('blockid');
      mask Callback storagetype: waijung_vdata_read_callback('storagetype');
      mask Display: text(0.05, 0.5, 'Buffer: c','ver','middle','hor','left');port_label('output',1,'D1(double)')
  Volatile Data Storage Read2 : S-Function  FunctionName=waijung_vdata_read  Parameters=storagename,varname,sampletime,sampletimestr,blockid,storagetype,storagetypestr  EnableBusSupport=off  mask(waijung_vdata_read){storagename=c, varname=VolatileDataStorage3_c, sampletime=-1, sampletimestr=0.01, blockid=VolatileDataStorageRead2, storagetype=double, storagetypestr=double}
      mask prompts: storagename "Storage Name"; varname "Variable name"; sampletime "Sample time (sec)"; sampletimestr "Compiled sample time (sec) in string"; storagetype "Data type"; storagetypestr "Data type string"
      mask help: This block implements read data from a buffer.
      mask init:
      | waijung_vdata_read_callback('init');
      mask Help: web(fullfile(waijungdocroot,'Volatile_Data_Storage_Read.htm'))
      mask TypeOptions storagename: condicion | c
      mask Callback storagename: waijung_vdata_read_callback('storagename');
      mask Callback varname: waijung_vdata_read_callback('varname');
      mask Callback sampletime: waijung_vdata_read_callback('sampletime');
      mask Callback sampletimestr: waijung_vdata_read_callback('sampletimestr');
      mask Callback blockid: waijung_vdata_read_callback('blockid');
      mask Callback storagetype: waijung_vdata_read_callback('storagetype');
      mask Display: text(0.05, 0.5, 'Buffer: c','ver','middle','hor','left');port_label('output',1,'D1(double)')
  Volatile Data Storage Read3 : S-Function  FunctionName=waijung_vdata_read  Parameters=storagename,varname,sampletime,sampletimestr,blockid,storagetype,storagetypestr  EnableBusSupport=off  mask(waijung_vdata_read){storagename=c, varname=VolatileDataStorage3_c, sampletime=-1, sampletimestr=0.01, blockid=VolatileDataStorageRead3, storagetype=double, storagetypestr=double}
      mask prompts: storagename "Storage Name"; varname "Variable name"; sampletime "Sample time (sec)"; sampletimestr "Compiled sample time (sec) in string"; storagetype "Data type"; storagetypestr "Data type string"
      mask help: This block implements read data from a buffer.
      mask init:
      | waijung_vdata_read_callback('init');
      mask Help: web(fullfile(waijungdocroot,'Volatile_Data_Storage_Read.htm'))
      mask TypeOptions storagename: condicion | c
      mask Callback storagename: waijung_vdata_read_callback('storagename');
      mask Callback varname: waijung_vdata_read_callback('varname');
      mask Callback sampletime: waijung_vdata_read_callback('sampletime');
      mask Callback sampletimestr: waijung_vdata_read_callback('sampletimestr');
      mask Callback blockid: waijung_vdata_read_callback('blockid');
      mask Callback storagetype: waijung_vdata_read_callback('storagetype');
      mask Display: text(0.05, 0.5, 'Buffer: c','ver','middle','hor','left');port_label('output',1,'D1(double)')
  Volatile Data Storage Read4 : S-Function  FunctionName=waijung_vdata_read  Parameters=storagename,varname,sampletime,sampletimestr,blockid,storagetype,storagetypestr  EnableBusSupport=off  mask(waijung_vdata_read){storagename=c, varname=VolatileDataStorage3_c, sampletime=-1, sampletimestr=0.01, blockid=VolatileDataStorageRead4, storagetype=double, storagetypestr=double}
      mask prompts: storagename "Storage Name"; varname "Variable name"; sampletime "Sample time (sec)"; sampletimestr "Compiled sample time (sec) in string"; storagetype "Data type"; storagetypestr "Data type string"
      mask help: This block implements read data from a buffer.
      mask init:
      | waijung_vdata_read_callback('init');
      mask Help: web(fullfile(waijungdocroot,'Volatile_Data_Storage_Read.htm'))
      mask TypeOptions storagename: condicion | c
      mask Callback storagename: waijung_vdata_read_callback('storagename');
      mask Callback varname: waijung_vdata_read_callback('varname');
      mask Callback sampletime: waijung_vdata_read_callback('sampletime');
      mask Callback sampletimestr: waijung_vdata_read_callback('sampletimestr');
      mask Callback blockid: waijung_vdata_read_callback('blockid');
      mask Callback storagetype: waijung_vdata_read_callback('storagetype');
      mask Display: text(0.05, 0.5, 'Buffer: c','ver','middle','hor','left');port_label('output',1,'D1(double)')
  Volatile Data Storage Read5 : S-Function  FunctionName=waijung_vdata_read  Parameters=storagename,varname,sampletime,sampletimestr,blockid,storagetype,storagetypestr  EnableBusSupport=off  mask(waijung_vdata_read){storagename=c, varname=VolatileDataStorage3_c, sampletime=-1, sampletimestr=0.01, blockid=VolatileDataStorageRead5, storagetype=double, storagetypestr=double}
      mask prompts: storagename "Storage Name"; varname "Variable name"; sampletime "Sample time (sec)"; sampletimestr "Compiled sample time (sec) in string"; storagetype "Data type"; storagetypestr "Data type string"
      mask help: This block implements read data from a buffer.
      mask init:
      | waijung_vdata_read_callback('init');
      mask Help: web(fullfile(waijungdocroot,'Volatile_Data_Storage_Read.htm'))
      mask TypeOptions storagename: condicion | c
      mask Callback storagename: waijung_vdata_read_callback('storagename');
      mask Callback varname: waijung_vdata_read_callback('varname');
      mask Callback sampletime: waijung_vdata_read_callback('sampletime');
      mask Callback sampletimestr: waijung_vdata_read_callback('sampletimestr');
      mask Callback blockid: waijung_vdata_read_callback('blockid');
      mask Callback storagetype: waijung_vdata_read_callback('storagetype');
      mask Display: text(0.05, 0.5, 'Buffer: c','ver','middle','hor','left');port_label('output',1,'D1(double)')
  Volatile Data Storage2 : S-Function  FunctionName=waijung_vdata_storage  Parameters=storagetype,storagename,initval,varname,buffersize,initvalstring,sampletime,sampletimestr,blockid,storagetypestr  EnableBusSupport=off  mask(waijung_vdata_storage){storagetype=double, storagename=condicion, initval=0, varname=VolatileDataStorage2_condicion, buffersize=64, initvalstring='', sampletime=-1, sampletimestr=0.01, blockid=VolatileDataStorage2, storagetypestr=double}
      mask prompts: storagetype "Storage Type"; storagename "Storage Name (must be a valid variable name)"; initval "Initial value (Apply at Power on Reset only)"; varname "Variable name"; buffersize "Size (bytes)"; initvalstring "Initial value (Apply at Power on Reset only)"; sampletime "Sample time (sec)"; sampletimestr "Compiled sample time (sec) in string"; storagetypestr "Type string"
      mask help: This block implements a volatile Data Storage.
      mask init:
      | waijung_vdata_storage_callback('init');
      mask Help: web(fullfile(waijungdocroot,'Volatile_Data_Storage.htm'))
      mask TypeOptions storagetype: double | single | uint32 | int32 | uint16 | int16 | uint8 | int8 | string
      mask Callback storagetype: waijung_vdata_storage_callback('storagetype');
      mask Callback storagename: waijung_vdata_storage_callback('storagename');
      mask Callback initval: waijung_vdata_storage_callback('initval');
      mask Callback varname: waijung_vdata_storage_callback('varname');
      mask Callback initvalstring: waijung_vdata_storage_callback('initvalstring');
      mask Callback sampletime: waijung_vdata_storage_callback('sampletime');
      mask Callback sampletimestr: waijung_vdata_storage_callback('sampletimestr');
      mask Callback blockid: waijung_vdata_storage_callback('blockid');
      mask Display: text(0.5, 0.5, '! Out of date','ver','middle','hor','center')
  Volatile Data Storage3 : S-Function  FunctionName=waijung_vdata_storage  Parameters=storagetype,storagename,initval,varname,buffersize,initvalstring,sampletime,sampletimestr,blockid,storagetypestr  EnableBusSupport=off  mask(waijung_vdata_storage){storagetype=double, storagename=c, initval=0, varname=VolatileDataStorage3_c, buffersize=64, initvalstring='', sampletime=-1, sampletimestr=0.01, blockid=VolatileDataStorage3, storagetypestr=double}
      mask prompts: storagetype "Storage Type"; storagename "Storage Name (must be a valid variable name)"; initval "Initial value (Apply at Power on Reset only)"; varname "Variable name"; buffersize "Size (bytes)"; initvalstring "Initial value (Apply at Power on Reset only)"; sampletime "Sample time (sec)"; sampletimestr "Compiled sample time (sec) in string"; storagetypestr "Type string"
      mask help: This block implements a volatile Data Storage.
      mask init:
      | waijung_vdata_storage_callback('init');
      mask Help: web(fullfile(waijungdocroot,'Volatile_Data_Storage.htm'))
      mask TypeOptions storagetype: double | single | uint32 | int32 | uint16 | int16 | uint8 | int8 | string
      mask Callback storagetype: waijung_vdata_storage_callback('storagetype');
      mask Callback storagename: waijung_vdata_storage_callback('storagename');
      mask Callback initval: waijung_vdata_storage_callback('initval');
      mask Callback varname: waijung_vdata_storage_callback('varname');
      mask Callback initvalstring: waijung_vdata_storage_callback('initvalstring');
      mask Callback sampletime: waijung_vdata_storage_callback('sampletime');
      mask Callback sampletimestr: waijung_vdata_storage_callback('sampletimestr');
      mask Callback blockid: waijung_vdata_storage_callback('blockid');
      mask Display: text(0.5, 0.5, '! Out of date','ver','middle','hor','center')
  wires:
  Merge6/1 -> Basic PWM/1
  Volatile Data Storage Read13/1 -> Compare To Constant/1
  Digital Input/2 -> Digital Output2/3, [Hb]
  Digital Input/3 -> Digital Output2/4, [Ha]
  Logical Operator3/1 -> Logical Operator1/2
  Digital Input/1 -> Digital Output2/2, [Hc]
  Compare To Constant/1 -> Enabled Subsystem2/Enable
  Logical Operator1/1 -> Enabled Subsystem1/Enable
  [Ha] -> Logical Operator1/1
  [Hb] -> Logical Operator3/1
  [Hc] -> Logical Operator2/1
  Logical Operator2/1 -> Logical Operator1/3
  Enabled Subsystem2/2(Out2) -> [Q6_1]
  Enabled Subsystem2/1(Out1) -> [Q5_1]
  Enabled Subsystem1/1(Out1) -> [Q3_1]
  Enabled Subsystem1/2(Out2) -> [Q4_1]
  Enabled Subsystem1/3(Out3) -> [Q1_1]
  Enabled Subsystem1/4(Out4) -> [Q2_1]
  [Q1_1] -> Merge6/1
  [Q1_2] -> Merge6/2
  [Q1_3] -> Merge6/3
  [Q1_4] -> Merge6/4
  [Q1_5] -> Merge6/5
  [Q1_6] -> Merge6/6
  Merge1/1 -> Basic PWM1/1
  [Q6_1] -> Merge1/1
  [Q6_2] -> Merge1/2
  [Q6_3] -> Merge1/3
  [Q6_4] -> Merge1/4
  [Q6_5] -> Merge1/5
  [Q6_6] -> Merge1/6
  Merge2/1 -> Basic PWM2/1
  [Q2_1] -> Merge2/1
  [Q2_2] -> Merge2/2
  [Q2_3] -> Merge2/3
  [Q2_4] -> Merge2/4
  [Q2_5] -> Merge2/5
  [Q2_6] -> Merge2/6
  Merge3/1 -> Basic PWM3/1
  [Q5_1] -> Merge3/1
  [Q5_2] -> Merge3/2
  [Q5_3] -> Merge3/3
  [Q5_4] -> Merge3/4
  [Q5_5] -> Merge3/5
  [Q5_6] -> Merge3/6
  Merge4/1 -> Basic PWM4/1
  [Q4_1] -> Merge4/1
  [Q4_2] -> Merge4/2
  [Q4_3] -> Merge4/3
  [Q4_4] -> Merge4/4
  [Q4_5] -> Merge4/5
  [Q4_6] -> Merge4/6
  Merge5/1 -> Basic PWM5/1
  [Q3_1] -> Merge5/1
  [Q3_2] -> Merge5/2
  [Q3_3] -> Merge5/3
  [Q3_4] -> Merge5/4
  [Q3_5] -> Merge5/5
  [Q3_6] -> Merge5/6
  Volatile Data Storage Read1/1 -> Compare To Constant1/1
  Logical Operator6/1 -> Logical Operator4/2
  Compare To Constant1/1 -> Enabled Subsystem4/Enable
  Logical Operator4/1 -> Enabled Subsystem3/Enable
  [Ha] -> Logical Operator4/1
  [Hb] -> Logical Operator6/1
  [Hc] -> Logical Operator4/3
  Enabled Subsystem4/2(Out2) -> [Q4_2]
  Enabled Subsystem4/1(Out1) -> [Q5_2]
  Enabled Subsystem3/1(Out1) -> [Q1_2]
  Enabled Subsystem3/2(Out2) -> [Q2_2]
  Enabled Subsystem3/3(Out3) -> [Q3_2]
  Enabled Subsystem3/4(Out4) -> [Q6_2]
  Volatile Data Storage Read2/1 -> Compare To Constant2/1
  Logical Operator8/1 -> Logical Operator5/2
  Compare To Constant2/1 -> Enabled Subsystem6/Enable
  Logical Operator5/1 -> Enabled Subsystem5/Enable
  [Hb] -> Logical Operator8/1
  [Hc] -> Logical Operator5/3
  Enabled Subsystem6/2(Out2) -> [Q4_3]
  Enabled Subsystem6/1(Out1) -> [Q3_3]
  Enabled Subsystem5/1(Out1) -> [Q1_3]
  Enabled Subsystem5/2(Out2) -> [Q5_3]
  Enabled Subsystem5/3(Out3) -> [Q6_3]
  Enabled Subsystem5/4(Out4) -> [Q2_3]
  [Ha] -> Logical Operator9/1
  Logical Operator9/1 -> Logical Operator5/1
  Volatile Data Storage Read3/1 -> Compare To Constant3/1
  [Hb] -> Logical Operator7/2
  Compare To Constant3/1 -> Enabled Subsystem8/Enable
  Logical Operator7/1 -> Enabled Subsystem7/Enable
  [Hc] -> Logical Operator7/3
  Enabled Subsystem8/2(Out2) -> [Q2_4]
  Enabled Subsystem8/1(Out1) -> [Q3_4]
  Enabled Subsystem7/1(Out1) -> [Q1_4]
  Enabled Subsystem7/2(Out2) -> [Q4_4]
  Enabled Subsystem7/3(Out3) -> [Q5_4]
  Enabled Subsystem7/4(Out4) -> [Q6_4]
  [Ha] -> Logical Operator11/1
  Logical Operator11/1 -> Logical Operator7/1
  Volatile Data Storage Read4/1 -> Compare To Constant4/1
  Compare To Constant4/1 -> Enabled Subsystem10/Enable
  Logical Operator10/1 -> Enabled Subsystem9/Enable
  Enabled Subsystem10/2(Out2) -> [Q2_5]
  Enabled Subsystem10/1(Out1) -> [Q1_5]
  Enabled Subsystem9/1(Out1) -> [Q6_5]
  Enabled Subsystem9/2(Out2) -> [Q5_5]
  Enabled Subsystem9/3(Out3) -> [Q3_5]
  Enabled Subsystem9/4(Out4) -> [Q4_5]
  Logical Operator13/1 -> Logical Operator10/1
  [Ha] -> Logical Operator13/1
  [Hc] -> Logical Operator12/1
  Logical Operator12/1 -> Logical Operator10/3
  [Hb] -> Logical Operator10/2
  Volatile Data Storage Read5/1 -> Compare To Constant5/1
  Compare To Constant5/1 -> Enabled Subsystem12/Enable
  Logical Operator14/1 -> Enabled Subsystem11/Enable
  [Hb] -> Logical Operator14/2
  Enabled Subsystem12/2(Out2) -> [Q6_6]
  Enabled Subsystem12/1(Out1) -> [Q1_6]
  Enabled Subsystem11/1(Out1) -> [Q2_6]
  Enabled Subsystem11/2(Out2) -> [Q3_6]
  Enabled Subsystem11/3(Out3) -> [Q4_6]
  Enabled Subsystem11/4(Out4) -> [Q5_6]
  [Ha] -> Logical Operator14/1
  Logical Operator16/1 -> Logical Operator14/3
  [Hc] -> Logical Operator16/1
  Regular ADC2/1 -> Gain/1
  Gain/1 -> Saturation/1
  Saturation/1 -> [setpoint], Sum/1
  [control] -> Enabled Subsystem2/1(In1)
  [control] -> Enabled Subsystem4/1(In1)
  [control] -> Enabled Subsystem6/1(In1)
  [control] -> Enabled Subsystem8/1(In1)
  [control] -> Enabled Subsystem10/1(In1)
  [control] -> Enabled Subsystem12/1(In1)
  Derivative1/1 -> SMC1/3(dX(t))
  [sensor] -> Sum/2, SMC1/2(x(t)), Derivative1/1
  Sum/1 -> SMC1/1(e(t))
  SMC1/1(Out1) -> [d], Saturation1/1
  Data Type Conversion/1 -> UART Tx/1
  PWM Capture/4 -> Data Type Conversion1/1
  [setpoint] -> "Data Type Conversion2 "/1
  "Data Type Conversion2 "/1 -> UART Tx/2
  Data Type Conversion2/1 -> UART Tx/3
  [control] -> Data Type Conversion2/1
  Saturation1/1 -> [control]
  Data Type Conversion1/1 -> Gain1/1
  Gain1/1 -> [sensor], Data Type Conversion/1
  Digital Input/4 -> Digital Output2/1
